simulink model "alfa"  (R2013b)
settings: Solver=ode45  StartTime=0.0  StopTime=10.0  RelTol=1e-3
undefined symbols (not defined in the file or in its folder): a, b
libraries: simulink x3
settings Model: Creator=Eduardo  LastModifiedBy=Eduardo

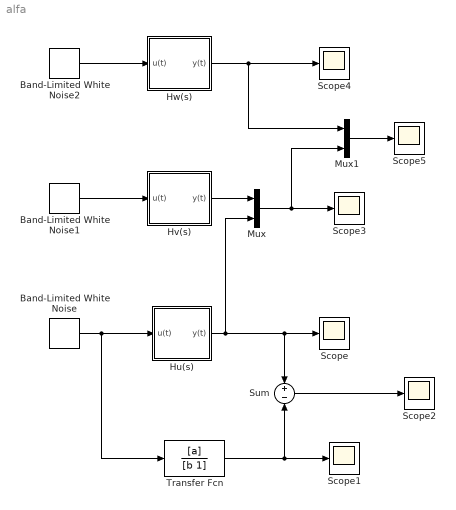
== system alfa ==
  Band-Limited White Noise : simulink/Sources/Band-Limited White Noise  Cov=[0.1]  Ts=0.1  seed=[23341]
  Band-Limited White Noise1 : simulink/Sources/Band-Limited White Noise  Cov=[0.1]  Ts=0.1  seed=[23348]
  Band-Limited White Noise2 : simulink/Sources/Band-Limited White Noise  Cov=[0.1]  Ts=0.1  seed=[21348]
  Hu(s) : Subsystem
  Hv(s) : Subsystem
  "Hw(s) " : Subsystem
  Mux : Mux  Inputs=2
  Mux1 : Mux  Inputs=2
  Scope{,1..5} (6 alike) : Scope
      Scope2 settings: SaveName=ScopeData2
      Scope3 settings: SaveName=ScopeData3
      Scope4 settings: SaveName=ScopeData4
      Scope5 settings: SaveName=ScopeData5
  Sum : Sum  Inputs=+|-
  Transfer Fcn : TransferFcn  Numerator=[a]  Denominator=[b 1]
  wires:
  Hu(s)/1(y(t)) -> Mux/2, Sum/1, Scope/1
  Transfer Fcn/1 -> Sum/2, Scope1/1
  Sum/1 -> Scope2/1
  Band-Limited White Noise/1 -> Hu(s)/1("u(t) "), Transfer Fcn/1
  Band-Limited White Noise1/1 -> Hv(s)/1("u(t) ")
  Hv(s)/1(y(t)) -> Mux/1
  Mux/1 -> Mux1/2, Scope3/1
  Band-Limited White Noise2/1 -> "Hw(s) "/1("u(t) ")
  "Hw(s) "/1(y(t)) -> Mux1/1, Scope4/1
  Mux1/1 -> Scope5/1

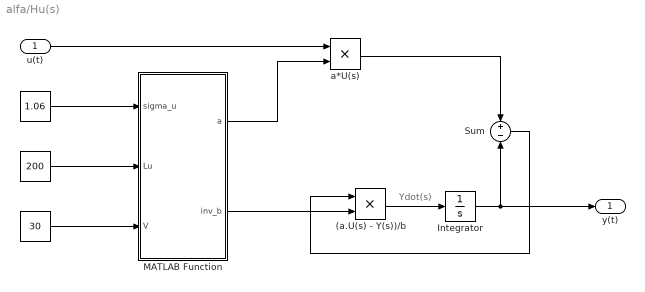
== system alfa/Hu(s) ==
  note: Ydot(s)
  "u(t) " : Inport
  " " : Constant  Value=1.06
  "  " : Constant  Value=200
  "   " : Constant  Value=30
  (a.U(s) - Y(s))/b : Product
  Integrator : Integrator
  MATLAB Function : MATLAB Function  TreatAsAtomicUnit=on
  Sum : Sum  Inputs=+|-
  a*U(s) : Product
  y(t) : Outport
  wires:
  MATLAB Function/1(a) -> a*U(s)/2
  Sum/1 -> (a.U(s) - Y(s))/b/1
  "   "/1 -> MATLAB Function/3(V)
  a*U(s)/1 -> Sum/1
  MATLAB Function/2(inv_b) -> (a.U(s) - Y(s))/b/2
  (a.U(s) - Y(s))/b/1 -> Integrator/1
  Integrator/1 -> y(t)/1, Sum/2
  " "/1 -> MATLAB Function/1(sigma_u)
  "  "/1 -> MATLAB Function/2(Lu)
  "u(t) "/1 -> a*U(s)/1

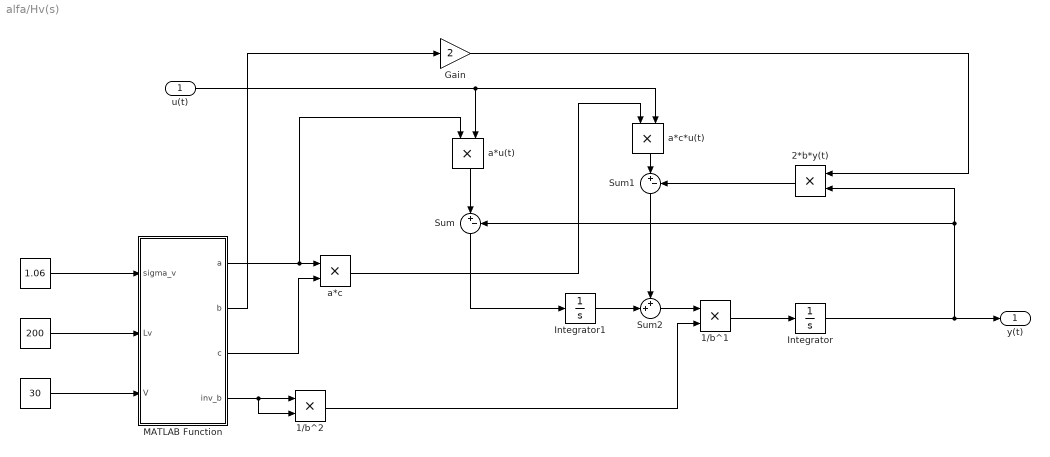
== system alfa/Hv(s) ==
  "u(t) " : Inport
  " " : Constant  Value=1.06
  "  " : Constant  Value=200
  "   " : Constant  Value=30
  1/b^1 : Product
  1/b^2 : Product
  2*b*y(t) : Product
  Gain : Gain  Gain=2
  Integrator : Integrator
  Integrator1 : Integrator
  MATLAB Function : MATLAB Function  TreatAsAtomicUnit=on
  Sum : Sum  Inputs=|+-
  Sum1 : Sum  Inputs=|+-
  Sum2 : Sum  Inputs=++|
  a*c : Product
  a*c*u(t) : Product
  a*u(t) : Product
  y(t) : Outport
  wires:
  "   "/1 -> MATLAB Function/3(V)
  " "/1 -> MATLAB Function/1(sigma_v)
  "  "/1 -> MATLAB Function/2(Lv)
  MATLAB Function/4(inv_b) -> 1/b^2/2, 1/b^2/1
  MATLAB Function/1(a) -> a*u(t)/1, a*c/1
  MATLAB Function/3(c) -> a*c/2
  "u(t) "/1 -> a*c*u(t)/2, a*u(t)/2
  a*u(t)/1 -> Sum/1
  Integrator/1 -> 2*b*y(t)/2, Sum/2, y(t)/1
  a*c/1 -> a*c*u(t)/1
  a*c*u(t)/1 -> Sum1/1
  MATLAB Function/2(b) -> Gain/1
  Gain/1 -> 2*b*y(t)/1
  2*b*y(t)/1 -> Sum1/2
  Sum/1 -> Integrator1/1
  Integrator1/1 -> Sum2/2
  Sum1/1 -> Sum2/1
  1/b^2/1 -> 1/b^1/2
  Sum2/1 -> 1/b^1/1
  1/b^1/1 -> Integrator/1

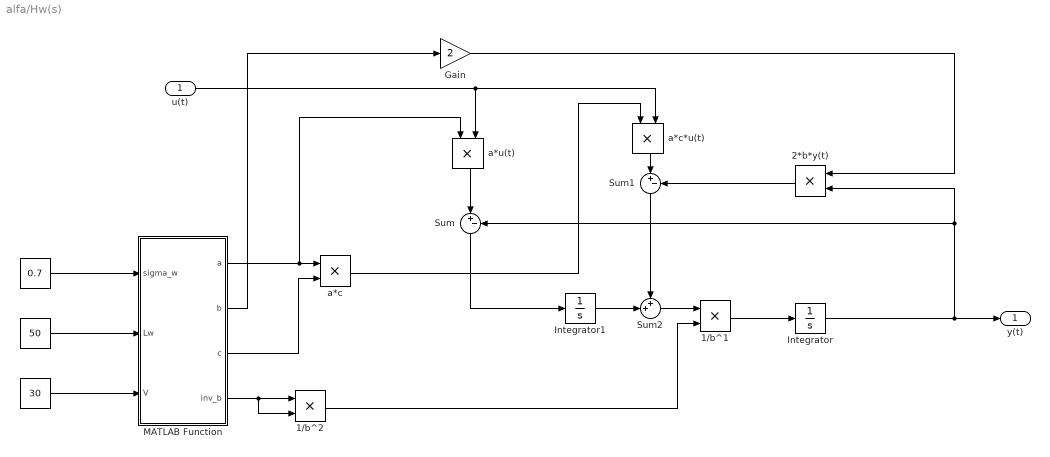
== system alfa/Hw(s)  ==
  "u(t) " : Inport
  " " : Constant  Value=0.7
  "  " : Constant  Value=50
  "   " : Constant  Value=30
  1/b^1 : Product
  1/b^2 : Product
  2*b*y(t) : Product
  Gain : Gain  Gain=2
  Integrator : Integrator
  Integrator1 : Integrator
  MATLAB Function : MATLAB Function  TreatAsAtomicUnit=on
  Sum : Sum  Inputs=|+-
  Sum1 : Sum  Inputs=|+-
  Sum2 : Sum  Inputs=++|
  a*c : Product
  a*c*u(t) : Product
  a*u(t) : Product
  y(t) : Outport
  wires:
  "   "/1 -> MATLAB Function/3(V)
  " "/1 -> MATLAB Function/1(sigma_w)
  "  "/1 -> MATLAB Function/2(Lw)
  MATLAB Function/4(inv_b) -> 1/b^2/2, 1/b^2/1
  MATLAB Function/1(a) -> a*u(t)/1, a*c/1
  MATLAB Function/3(c) -> a*c/2
  "u(t) "/1 -> a*c*u(t)/2, a*u(t)/2
  a*u(t)/1 -> Sum/1
  Integrator/1 -> 2*b*y(t)/2, Sum/2, y(t)/1
  a*c/1 -> a*c*u(t)/1
  a*c*u(t)/1 -> Sum1/1
  MATLAB Function/2(b) -> Gain/1
  Gain/1 -> 2*b*y(t)/1
  2*b*y(t)/1 -> Sum1/2
  Sum/1 -> Integrator1/1
  Integrator1/1 -> Sum2/2
  Sum1/1 -> Sum2/1
  1/b^2/1 -> 1/b^1/2
  Sum2/1 -> 1/b^1/1
  1/b^1/1 -> Integrator/1

== matlab function alfa/Hv(s)/MATLAB Function ==
  data: sigma_v input; a output; b output; c output; Lv input; V input; inv_b output
function [a, b, c, inv_b] = fcn(sigma_v, Lv, V)

a = sigma_v*sqrt(Lv/(pi*V));
b = Lv/V;
c = sqrt(3)*Lv/V;
inv_b = 1/b;

end

== matlab function alfa/Hu(s)/MATLAB Function ==
  data: sigma_u input; a output; Lu input; V input; inv_b output
function [a, inv_b] = fcn(sigma_u, Lu, V)

a = sigma_u*sqrt(2*Lu/(pi*V));
b = Lu/V;
inv_b = 1/b;

end

== matlab function alfa/Hw(s) /MATLAB Function ==
  data: sigma_w input; a output; b output; c output; Lw input; V input; inv_b output
function [a, b, c, inv_b] = fcn(sigma_w, Lw, V)

a = sigma_w*sqrt(Lw/(pi*V));
b = Lw/V;
c = sqrt(3)*Lw/V;
inv_b = 1/b;

end
